simulink model "ShastaSimulink"  (R2025b)
settings: Solver=VariableStepAuto  StartTime=0.0  StopTime=80  RelTol=1e-3
model workspace (MAT data in the model file):
  Cd_body = 0.733
  Sig = Simulink.Signal
  Sig.Dimensions = -1
  Sig.DimensionsMode = 'auto'
  Sig.Complexity = 'auto'
  Sig.SampleTime = -1
  Sig.SamplingMode = 'auto'
  Sig.DataType = 'auto'
  Var = 0
  mass = 0.964
settings Model: Creator=lawtonskaling  LastModifiedBy=2015k

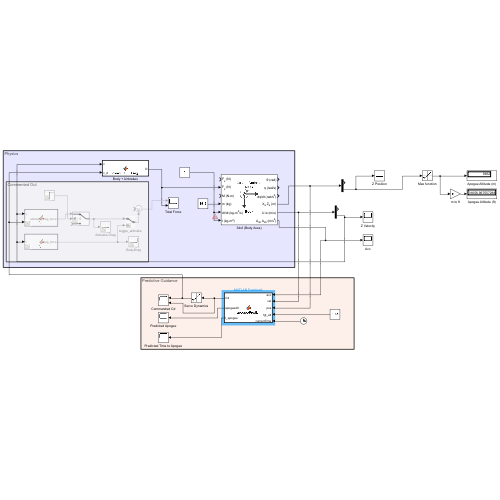
[thumbnail: Simulink's stored preview of the top-level diagram]
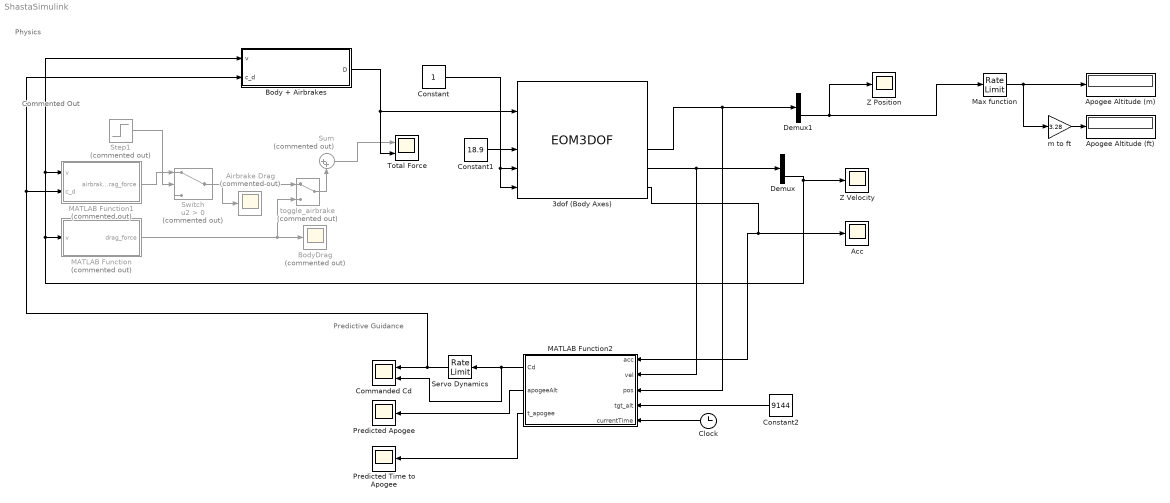
== system ShastaSimulink ==
  note: Commented Out
  note: Predictive Guidance
  note: Physics
  3dof (Body Axes) : EOM3DOF  mtype=Custom Variable  v_ini=350  alpha_ini=90  pos_ini=[0 5849.11]  mass=mass  g=-9.81
  Acc : Scope
  Airbrake Drag : Scope  Commented=on
      settings: ActiveDisplayYMinimum=-528.36647  ActiveDisplayYMaximum=112.77411  DataLoggingVariableName=ScopeData3
  Apogee Altitude (ft) : Display
  Apogee Altitude (m) : Display
  Body + Airbrakes : MATLAB Function  TreatAsAtomicUnit=on
  BodyDrag : Scope  Commented=on
      settings: ActiveDisplayYMinimum=-168.21044  ActiveDisplayYMaximum=34.07992
  Clock : Clock
  Commanded Cd : Scope  NumInputPorts=2
      settings: DataLoggingVariableName=ScopeData8
  Constant : Constant
  Constant1 : Constant  Value=18.9
  Constant2 : Constant  Value=9144
  Demux : Demux  Outputs=2
  Demux1 : Demux  Outputs=2
  MATLAB Function : MATLAB Function  Commented=on  TreatAsAtomicUnit=on
  MATLAB Function1 : MATLAB Function  Commented=on  TreatAsAtomicUnit=on
  MATLAB Function2 : MATLAB Function  TreatAsAtomicUnit=on
  Max function : RateLimiter  RisingSlewLimit=inf  FallingSlewLimit=0  SampleTimeMode=inherited
  Predicted Apogee : Scope
      settings: DataLoggingVariableName=ScopeData7
  Predicted Time to Apogee : Scope
      settings: DataLoggingVariableName=ScopeData6
  Servo Dynamics : RateLimiter  RisingSlewLimit=1.2  FallingSlewLimit=-1.2  SampleTimeMode=inherited
  Step1 : Step  Commented=on  SampleTime=0
  Sum : Sum  Commented=on  Inputs=|++
  Switch : Switch  Commented=on  Criteria=u2 > Threshold  SaturateOnIntegerOverflow=off  InputSameDT=off
  Total Force : Scope  NumInputPorts=2
      settings: ActiveDisplayYMinimum=-3794.7564502256746  ActiveDisplayYMaximum=5970.6732514977966  DataLoggingVariableName=ScopeData4
  Z Position : Scope
      settings: ActiveDisplayYMinimum=-1  ActiveDisplayYMaximum=1  DataLoggingVariableName=ScopeData5
  Z Velocity : Scope
      settings: ActiveDisplayYMinimum=-31.73523  ActiveDisplayYMaximum=201.30688  DataLoggingVariableName=ScopeData2
  m to ft : Gain  Gain=3.28
  toggle_airbrake : ManualSwitch  Commented=on
  wires:
  Sum/1 -> Total Force/1
  MATLAB Function/1(drag_force) -> BodyDrag/1, toggle_airbrake/2
  3dof (Body Axes)/5 -> Demux/1, MATLAB Function2/2(vel)
  Demux/2 -> Z Velocity/1, MATLAB Function1/1(v), Body + Airbrakes/1(v), MATLAB Function/1(v)
  3dof (Body Axes)/4 -> Demux1/1, MATLAB Function2/3(pos)
  Demux1/2 -> Z Position/1, Max function/1
  Max function/1 -> m to ft/1, Apogee Altitude (m)/1
  toggle_airbrake/1 -> Sum/2
  Switch/1 -> toggle_airbrake/1, Airbrake Drag/1
  Step1/1 -> Switch/2
  MATLAB Function1/1(airbrake_drag_force) -> Switch/1
  m to ft/1 -> Apogee Altitude (ft)/1
  Constant/1 -> 3dof (Body Axes)/6, 3dof (Body Axes)/5
  Constant1/1 -> 3dof (Body Axes)/4
  3dof (Body Axes)/6 -> MATLAB Function2/1(acc), Acc/1
  MATLAB Function2/1(Cd) -> Commanded Cd/2, Servo Dynamics/1
  Servo Dynamics/1 -> MATLAB Function1/2(c_d), Body + Airbrakes/2(c_d), Commanded Cd/1
  MATLAB Function2/3(t_apogee) -> Predicted Time to Apogee/1
  MATLAB Function2/2(apogeeAlt) -> Predicted Apogee/1
  Clock/1 -> MATLAB Function2/5(currentTime)
  Body + Airbrakes/1(D) -> Total Force/2, 3dof (Body Axes)/2
  Constant2/1 -> MATLAB Function2/4(tgt_alt)

== matlab function ShastaSimulink/MATLAB Function1 ==
  data: v input; airbrake_drag_force output; c_d input
function airbrake_drag_force = fcn(v, c_d) % m/s

rho = 0.59; %kg / m^3
%A_ref = (3 * 25 * 30)/1000^2; %Shasta 
A_ref = (4 * 50 * 60)/1000^2; % m^2

body_drag = 0.5*rho*v.^2*c_d*A_ref; % N

airbrake_drag_force = body_drag .* sign(v) * -1;

== matlab function ShastaSimulink/MATLAB Function ==
  data: v input; drag_force output
function drag_force = fcn(v)

rho = 0.59; %kg / m^3
% A_ref = 3505 / 1000^2;% Shasta
% c_d = 0.733; % Shasta

c_d = 0.632; %IREC
A_ref = 8107 / 1000^2; %IREC

body_drag = 0.5*rho*v.^2*c_d*A_ref;

drag_force = body_drag .* sign(v) * -1;

== matlab function ShastaSimulink/MATLAB Function2 ==
  data: acc input; Cd output; vel input; pos input; tgt_alt input; currentTime input; apogeeAlt output; t_apogee output
function [Cd, apogeeAlt, t_apogee] = apogeePredict(acc, vel, pos, tgt_alt, currentTime)
    % Inputs:
    % acc - Acceleration vector: x and z accelerations
    % vel - Velocity vector: [U, W]. Only care abt W (z-velocity)
    % pos - Position vector: same as above
    % tgt_alt - target altitude (m)
    % currentTime - Current time in secs from launch

    apogeeTgt = tgt_alt;
    currentAlt = pos(2);
    currentZvel = vel(2);
    currentZacc = acc(2);

    rho = 0.59; %kg / m^3
    A = 8107 / 1000^2; %IREC, m^2, cross-sectional area of rocket;
    Cd_clean = 0.632; % Cd w no airbrakes
    m = 18.9; % kg
    v_sim = currentZvel;
    alt_sim = currentAlt;
    t = currentTime;
    deltaT = 0.01; % timestep of sims (s)
    apogeeAlt = 0;
    t_apogee = 0; 

    if(currentZacc > 0)
        Cd = Cd_clean;
        return;
    end

    % test various drag coeffs    
    for c = 1:15
        % predictive apogee modeling
        Cd_sim = Cd_clean + c*0.02;

        % TODO: Replace w RK45 HERE!!!
        % t0 = 0;
        % tf = 80;
        % tspan = [t0, tf]

        % Explicit Euler Method
        for i = 1:3000
            % drag equation: TODO make A a function!!!
            F = -0.5 * Cd_sim * rho * A * (v_sim^2) - 9.81*m;

            % Explicit Euler integration -> replace w rk45
            a_sim = F/m;
            v_sim = v_sim + a_sim * deltaT;
            t = t + deltaT;

            % apogee check: if Zvel <  0
            if v_sim < 0
                apogeeAlt = alt_sim;
                t_apogee = t;
                break;
            end
        end
        % if below target alt, choose as Cd
        Cd = Cd_sim;
        if apogeeAlt < apogeeTgt
            break;
        end
    end

== matlab function ShastaSimulink/Body + Airbrakes ==
  data: v input; D output; c_d input
function D = computeFullDrag(v, c_d) % m/s

rho = 0.59; %kg / m^3
% A_ref = 3505 / 1000^2;% Shasta
% c_d = 0.733; % Shasta

% c_d = 0.632; %IREC
A_ref_body = 8107 / 1000^2; %IREC

A_ref_ab = (4 * 50 * 60)/1000^2; % m^2

% body_drag = 0.5*rho*v.^2*c_d*A_ref * sign(v) * -1;
D = 0.5 * rho * v.^2 * c_d * A_ref_body * sign(v) * -1;
